simulink subsystem "OutputMotores"  (R2021b)
settings: Solver=VariableStepAuto  StartTime=0.0  StopTime=10.0  RelTol=1e-3
libraries: arduinolib x4
settings Model: Creator=yo  LastModifiedBy=yo

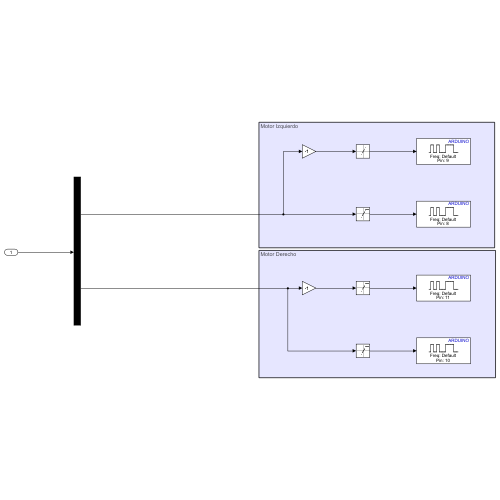
[thumbnail: Simulink's stored preview of the top-level diagram]
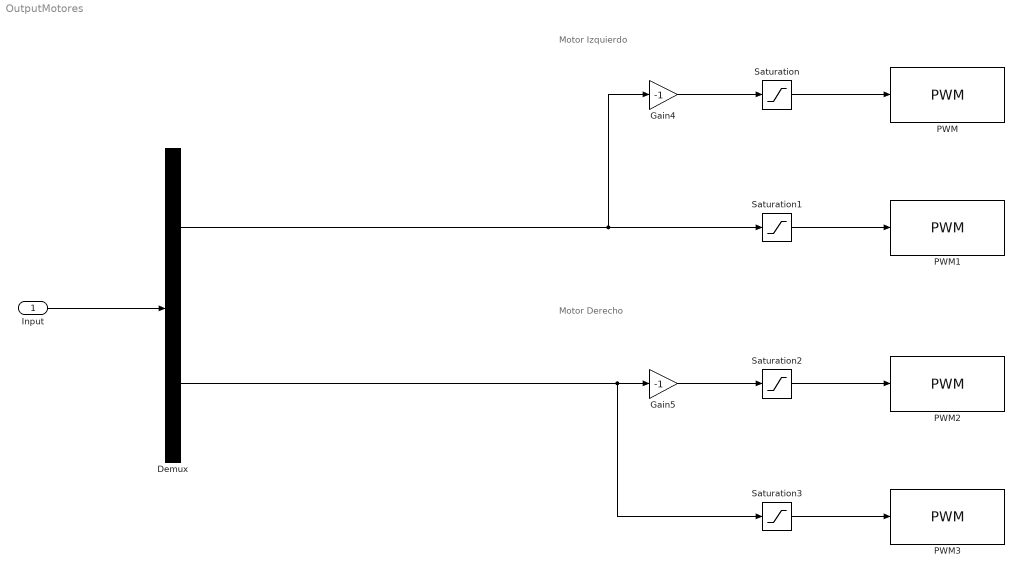
== system OutputMotores ==
  note: Motor Derecho
  note: Motor Izquierdo
  Input : Inport
  Demux : Demux  Outputs=2
  Gain4 : Gain  Gain=-1
  Gain5 : Gain  Gain=-1
  PWM : arduinolib/PWM  pinNumber=8  frequencyType=Default  desiredFrequency=490.2  achievableFrequency=490.2
  PWM1 : arduinolib/PWM  pinNumber=9  frequencyType=Default  desiredFrequency=490.2  achievableFrequency=490.2
  PWM2 : arduinolib/PWM  pinNumber=10  frequencyType=Default  desiredFrequency=490.2  achievableFrequency=490.2
  PWM3 : arduinolib/PWM  pinNumber=11  frequencyType=Default  desiredFrequency=490.2  achievableFrequency=490.2
  Saturation{,1..3} (4 alike) : Saturate  UpperLimit=255  LowerLimit=0
  wires:
  Demux/1 -> Gain4/1, Saturation1/1
  Input/1 -> Demux/1
  Saturation/1 -> PWM/1
  Saturation3/1 -> PWM3/1
  Gain4/1 -> Saturation/1
  Gain5/1 -> Saturation2/1
  Saturation2/1 -> PWM2/1
  Demux/2 -> Saturation3/1, Gain5/1
  Saturation1/1 -> PWM1/1
